simulink model "are_dre_sim"  (R2025b)
settings: Solver=VariableStepAuto  StartTime=0.0  StopTime=10  RelTol=1e-3
values from neighbouring files (symbols this model uses):
  A = [1 -2 ... (first row only)    [ARE_DRE_analysis.m]
  B = [0 ... (first row only)    [ARE_DRE_analysis.m]
  P = care(A,B,Q,R,S)    [ARE_DRE_analysis.m]
  R = 1    [ARE_DRE_analysis.m]
libraries: matrix_library x1
settings Model: Creator=Armando  LastModifiedBy=Armando

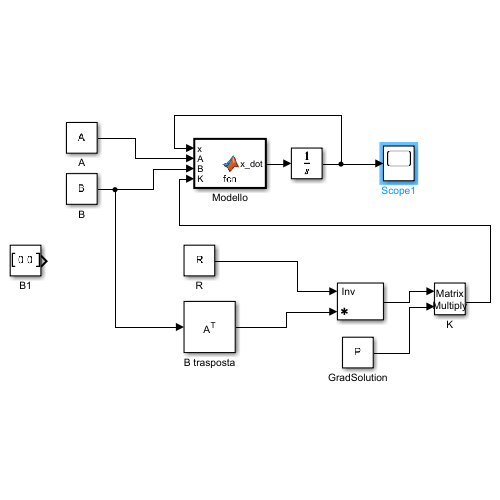
[thumbnail: Simulink's stored preview of the top-level diagram]
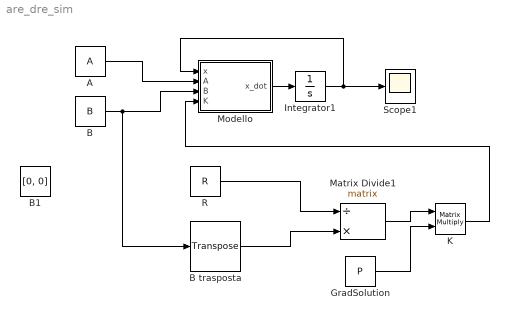
== system are_dre_sim ==
  A : Constant  Value=A
  B : Constant  Value=B
  B trasposta : matrix_library/Transpose
  B1 : Constant  Value=[0, 0]  VectorParams1D=off
  GradSolution : Constant  Value=P
  Integrator1 : Integrator  InitialCondition=[20;20]
  K : Product  Multiplication=Matrix(*)
  Matrix Divide1 : Product  Inputs=/*  Multiplication=Matrix(*)
  Modello : MATLAB Function  TreatAsAtomicUnit=on
  R : Constant  Value=R  VectorParams1D=off
  Scope1 : Scope
      settings: ActiveDisplayYMinimum=-25.4325397309699  ActiveDisplayYMaximum=25.048059970107765
  wires:
  GradSolution/1 -> K/2
  R/1 -> Matrix Divide1/1
  Integrator1/1 -> Scope1/1, Modello/1(x)
  B trasposta/1 -> Matrix Divide1/2
  B/1 -> B trasposta/1, Modello/3(B)
  A/1 -> Modello/2(A)
  Matrix Divide1/1 -> K/1
  Modello/1(x_dot) -> Integrator1/1
  K/1 -> Modello/4(K)

== matlab function are_dre_sim/Modello ==
  data: x input; A input; x_dot output; B input; K input
function x_dot = fcn(x,A,B,K)
    x_dot = linear_system(x,A,B,K);
end
